simulink model "model2v4"  (R2020b)
settings: Solver=VariableStepAuto  StartTime=0.0  StopTime=10.0  RelTol=1e-3
settings Model: Creator=dkravchenko  LastModifiedBy=dkravchenko

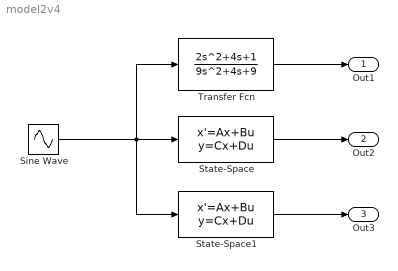
== system model2v4 ==
  Sine Wave : Sin  Amplitude=0  Bias=1  Frequency=0  SampleTime=0
  State-Space : StateSpace  A=[0 1 0; 0 0 1; -9 -4 -9]  B=[0; 0; 1]  C=[1 4 2]  D=0  InitialCondition=0
  State-Space1 : StateSpace  A=[0 0 -9; 1 0 -4; 0 1 -9]  B=[1; 4; 2]  C=[0 0 1]  D=0  InitialCondition=0
  Transfer Fcn : TransferFcn  Numerator=[2 4 1]  Denominator=[9 4 9]
  Out1 : Outport
  Out2 : Outport  Port=2
  Out3 : Outport  Port=3
  wires:
  Sine Wave/1 -> State-Space1/1, Transfer Fcn/1, State-Space/1
  Transfer Fcn/1 -> Out1/1
  State-Space/1 -> Out2/1
  State-Space1/1 -> Out3/1
